simulink model "mrefrobotarm_modified_previous_y_previous_u_previous_ref_Thao"  (R2018b)
settings: Solver=FixedStepAuto  StartTime=0.0  StopTime=10  RelTol=1e-3  AbsTol=1e-6
undefined symbols (not defined in the file or in its folder): sfunxy2
libraries: neural x668, simulink x1
(part 17 of 21)

== system mrefrobotarm_modified_previous_y_previous_u_previous_ref_Thao/trimmed_cex/Layer 2/LW{2,1} ==
  "ad{2,1}" : Inport  PortDimensions=40
      mask Display: e = 0.06;c1 = [120 230 180]/255;c2 = ([120 230 180]+0)/(256+128);c3 = ([120 230 180]+128)/(256+128);patch([0 1 1 0],[0 0 1 1],c1);patch([0 1 1 1-e 1-e 0+e],[0 0 1 1-e 0+e 0+e],c2);patch([0 0 1 1-e 0+e 0+e],[0 1 1 1-e 1-e 0+e],c3);plot([0 1 1 0 0],[0 0 1 1 0]);
  "IW{2,1}(1,:)'" : Constant  Value=[-0.1197125311373569422901397274472401477396488189697265625;0.93141849603577753224925572794745676219463348388671875;0.004886359461366405858295802744351021829061210155487060546875;-0.1512746681304759643893476095399819314479827880859375;-0.167852357976244148662914312808425165712833404541015625;0.10006780281716527725155430061931838281452655792236328125;0.10181621299721650697467367763238144107162952423095703125;0.309725252258556238427189555295626632869243621826171875;-0.02933411195067354981791396539847482927143573760986328125;-0.0152198482308951478503278309517554589547216892242431640625;-0.330145430668005668284337161821895278990268707275390625;0.076789053257603046009904801394441165030002593994140625;-0.375398541974394428510919397012912668287754058837890625;0.382117841615298547974788334613549523055553436279296875;0.2201335081328267551104005406159558333456516265869140625;-0.13146013321116478689276618752046488225460052490234375;-0.0249539477614627684676218422055171686224639415740966796875;0.402936988611822866079847926812362857162952423095703125;-0.011171185980911817192673396448299172334372997283935546875;0.1036892109939195893986152441357262432575225830078125;-0.01468148224949680953621555801191789214499294757843017578125;-0.0351746242361976324541927851896616630256175994873046875;-0.45375320694342102800789007233106531202793121337890625;0.025604358260133124047808195200559566728770732879638671875;0.1991726441753766396747238331954577006399631500244140625;-0.19735600633120575775336646984214894473552703857421875;-0.0906818380815199720501595948007889091968536376953125;0.415050002351403268807672475304570980370044708251953125;0.2385038498913788773680977328695007599890232086181640625;0.053659262377953688416543087669197120703756809234619140625;-0.00831153444230189712704781612728766049258410930633544921875;-0.279703049728368624560204125373275019228458404541015625;-0.122675859787673591227985525620169937610626220703125;0.12231550321479693621551376736533711664378643035888671875;0.40279223208026382341273574638762511312961578369140625;0.398579712933626983950574640402919612824916839599609375;-0.0806627151487938343077388481106027029454708099365234375;0.262880682610419580402805195262772031128406524658203125;-0.73968018525003476071333352592773735523223876953125;-0.5854281940437520148634575889445841312408447265625]
      mask Display: e = 0.06;c1 = [120 150 230]/255;c2 = ([120 150 230]+0)/383;c3 = ([120 150 230]+128)/383;patch([0 1 1 0],[0 0 1 1],c1);patch([0 1 1 1-e 1-e 0+e],[0 0 1 1-e 0+e 0+e],c2);patch([0 0 1 1-e 0+e 0+e],[0 1 1 1-e 1-e 0+e],c3);plot([0 1 1 0 0],[0 0 1 1 0]);disp('weights');
  Mux : Mux  Inputs=1
      mask Display: e = 0.06;c1 = [120 150 230]/255;c2 = ([120 150 230]+0)/383;c3 = ([120 150 230]+128)/383;patch([0 1 1 0],[0 0 1 1],c1);patch([0 1 1 1-e 1-e 0+e],[0 0 1 1-e 0+e 0+e],c2);patch([0 0 1 1-e 0+e 0+e],[0 1 1 1-e 1-e 0+e],c3);plot([0 1 1 0 0],[0 0 1 1 0]);disp('Mux');
  dotprod1 : neural/Weight Functions/dotprod
  "lz{2,1}" : Outport
      mask Display: e = 0.06;c1 = [120 230 180]/255;c2 = ([120 230 180]+0)/(256+128);c3 = ([120 230 180]+128)/(256+128);patch([0 1 1 0],[0 0 1 1],c1);patch([0 1 1 1-e 1-e 0+e],[0 0 1 1-e 0+e 0+e],c2);patch([0 0 1 1-e 0+e 0+e],[0 1 1 1-e 1-e 0+e],c3);plot([0 1 1 0 0],[0 0 1 1 0]);
  wires:
  "IW{2,1}(1,:)'"/1 -> dotprod1/1
  "ad{2,1}"/1 -> dotprod1/2
  dotprod1/1 -> Mux/1
  Mux/1 -> "lz{2,1}"/1

== system mrefrobotarm_modified_previous_y_previous_u_previous_ref_Thao/trimmed_cex_2/Layer 1/Delays 1 ==
  "p{1}" : Inport  PortDimensions=10
      mask Display: e = 0.06;c1 = [120 230 180]/255;c2 = ([120 230 180]+0)/(256+128);c3 = ([120 230 180]+128)/(256+128);patch([0 1 1 0],[0 0 1 1],c1);patch([0 1 1 1-e 1-e 0+e],[0 0 1 1-e 0+e 0+e],c2);patch([0 0 1 1-e 0+e 0+e],[0 1 1 1-e 1-e 0+e],c3);plot([0 1 1 0 0],[0 0 1 1 0]);
  mux : Mux  Inputs=1
      mask Display: e = 0.06;c1 = [120 150 230]/255;c2 = ([120 150 230]+0)/383;c3 = ([120 150 230]+128)/383;patch([0 1 1 0],[0 0 1 1],c1);patch([0 1 1 1-e 1-e 0+e],[0 0 1 1-e 0+e 0+e],c2);patch([0 0 1 1-e 0+e 0+e],[0 1 1 1-e 1-e 0+e],c3);plot([0 1 1 0 0],[0 0 1 1 0]);disp('Mux')
  "pd{1,1}" : Outport
      mask Display: e = 0.06;c1 = [120 230 180]/255;c2 = ([120 230 180]+0)/(256+128);c3 = ([120 230 180]+128)/(256+128);patch([0 1 1 0],[0 0 1 1],c1);patch([0 1 1 1-e 1-e 0+e],[0 0 1 1-e 0+e 0+e],c2);patch([0 0 1 1-e 0+e 0+e],[0 1 1 1-e 1-e 0+e],c3);plot([0 1 1 0 0],[0 0 1 1 0]);
  wires:
  "p{1}"/1 -> mux/1
  mux/1 -> "pd{1,1}"/1

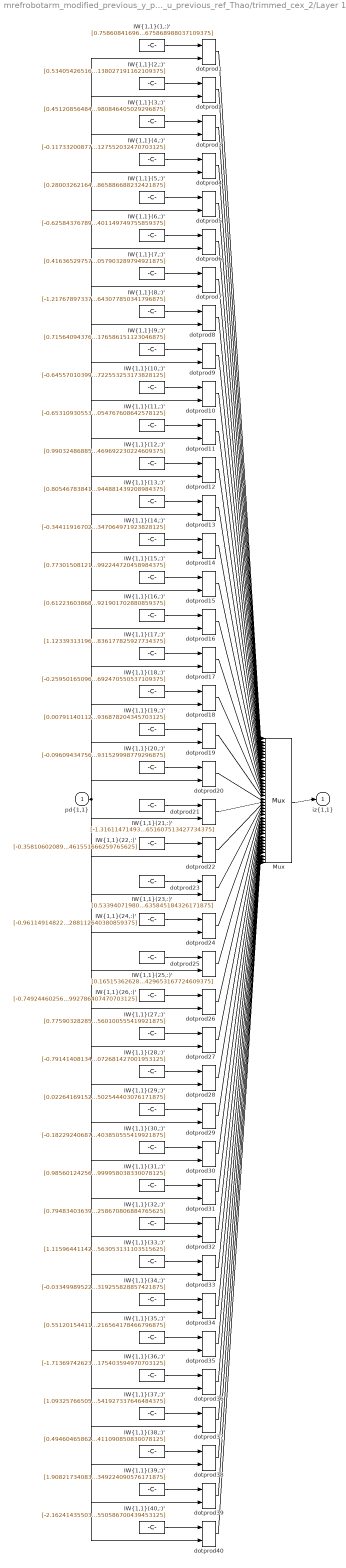
== system mrefrobotarm_modified_previous_y_previous_u_previous_ref_Thao/trimmed_cex_2/Layer 1/IW{1,1} ==
  "pd{1,1}" : Inport  PortDimensions=10
      mask Display: e = 0.06;c1 = [120 230 180]/255;c2 = ([120 230 180]+0)/(256+128);c3 = ([120 230 180]+128)/(256+128);patch([0 1 1 0],[0 0 1 1],c1);patch([0 1 1 1-e 1-e 0+e],[0 0 1 1-e 0+e 0+e],c2);patch([0 0 1 1-e 0+e 0+e],[0 1 1 1-e 1-e 0+e],c3);plot([0 1 1 0 0],[0 0 1 1 0]);
  "IW{1,1}(1,:)'" : Constant  Value=[0.7586084169638720453576752333901822566986083984375;0.64065528016229933427894138731062412261962890625;0.39576859169533984417199690142297185957431793212890625;0.67974231073814495029949966919957660138607025146484375;-0.8322839682529779015141002673772163689136505126953125;1.2325906050418289350290024231071583926677703857421875;-0.6476296846957207975492565310560166835784912109375;0.69513830019254607694989545052521862089633941650390625;0.362255404130632341352935554823488928377628326416015625;-0.83785018450818815605174449956393800675868988037109375]
      mask Display: e = 0.06;c1 = [120 150 230]/255;c2 = ([120 150 230]+0)/383;c3 = ([120 150 230]+128)/383;patch([0 1 1 0],[0 0 1 1],c1);patch([0 1 1 1-e 1-e 0+e],[0 0 1 1-e 0+e 0+e],c2);patch([0 0 1 1-e 0+e 0+e],[0 1 1 1-e 1-e 0+e],c3);plot([0 1 1 0 0],[0 0 1 1 0]);disp('Weights');
  "IW{1,1}(10,:)'" : Constant  Value=[-0.6455701039951160513652439476572908461093902587890625;0.6062395162995362074553895581630058586597442626953125;0.0841095892027095837217842699828906916081905364990234375;0.8395936116299094198467400929075665771961212158203125;-1.933433434291257579928924315026961266994476318359375;0.4699855661060308165133392321877181529998779296875;-1.3687077398461326982470609436859376728534698486328125;-0.1904722786551377999852974198802257888019084930419921875;0.326755886468258427424160572627442888915538787841796875;0.05237510702870014356324901427797158248722553253173828125]
      mask Display: e = 0.06;c1 = [120 150 230]/255;c2 = ([120 150 230]+0)/383;c3 = ([120 150 230]+128)/383;patch([0 1 1 0],[0 0 1 1],c1);patch([0 1 1 1-e 1-e 0+e],[0 0 1 1-e 0+e 0+e],c2);patch([0 0 1 1-e 0+e 0+e],[0 1 1 1-e 1-e 0+e],c3);plot([0 1 1 0 0],[0 0 1 1 0]);disp('Weights');
  "IW{1,1}(11,:)'" : Constant  Value=[-0.653109305534881112720313467434607446193695068359375;-0.63694471380195094578624548375955782830715179443359375;-0.66364616346480886921455066840280778706073760986328125;-1.5467933591431208828481658201781101524829864501953125;-0.953707704414698209660627981065772473812103271484375;0.016251165743796869289639062117203138768672943115234375;0.85764033268903105966529665238340385258197784423828125;-1.018200094286096923923423673841170966625213623046875;-1.006272936957347763353709524380974471569061279296875;-0.426306299052561066265099043448572047054767608642578125]
      mask Display: e = 0.06;c1 = [120 150 230]/255;c2 = ([120 150 230]+0)/383;c3 = ([120 150 230]+128)/383;patch([0 1 1 0],[0 0 1 1],c1);patch([0 1 1 1-e 1-e 0+e],[0 0 1 1-e 0+e 0+e],c2);patch([0 0 1 1-e 0+e 0+e],[0 1 1 1-e 1-e 0+e],c3);plot([0 1 1 0 0],[0 0 1 1 0]);disp('Weights');
  "IW{1,1}(12,:)'" : Constant  Value=[0.99032486885737236459448240566416643559932708740234375;-0.4064937633482277323793141476926393806934356689453125;-0.0653081845473883759733979559314320795238018035888671875;0.1267302228411903985971775910002179443836212158203125;-0.881843841858767074626257453928701579570770263671875;-0.062937554661245787013257313446956686675548553466796875;0.30167392474683563108328598900698125362396240234375;1.0408159785445139089432586843031458556652069091796875;-0.414501383489728036924049092704080976545810699462890625;-0.04337409273136037801688047466086572967469692230224609375]
      mask Display: e = 0.06;c1 = [120 150 230]/255;c2 = ([120 150 230]+0)/383;c3 = ([120 150 230]+128)/383;patch([0 1 1 0],[0 0 1 1],c1);patch([0 1 1 1-e 1-e 0+e],[0 0 1 1-e 0+e 0+e],c2);patch([0 0 1 1-e 0+e 0+e],[0 1 1 1-e 1-e 0+e],c3);plot([0 1 1 0 0],[0 0 1 1 0]);disp('Weights');
  "IW{1,1}(13,:)'" : Constant  Value=[0.80546783841772884304788249210105277597904205322265625;-0.0989022459644864071481862310974975116550922393798828125;-0.257406546599342422876333102976786904036998748779296875;-0.463638060984846667178516099738772027194499969482421875;0.118607183685509876003294493784778751432895660400390625;-1.064843433515526793797789650852791965007781982421875;-0.52909856619164463698012923487112857401371002197265625;-0.336660800704824236806445014735800214111804962158203125;-0.1735126677730877420291477619684883393347263336181640625;0.5562205162348961007268144385307095944881439208984375]
      mask Display: e = 0.06;c1 = [120 150 230]/255;c2 = ([120 150 230]+0)/383;c3 = ([120 150 230]+128)/383;patch([0 1 1 0],[0 0 1 1],c1);patch([0 1 1 1-e 1-e 0+e],[0 0 1 1-e 0+e 0+e],c2);patch([0 0 1 1-e 0+e 0+e],[0 1 1 1-e 1-e 0+e],c3);plot([0 1 1 0 0],[0 0 1 1 0]);disp('Weights');
  "IW{1,1}(14,:)'" : Constant  Value=[-0.344119167029077299702066738973371684551239013671875;-0.9444939814500035168975955457426607608795166015625;1.21324822037746482550346627249382436275482177734375;0.50228838522351237916296895491541363298892974853515625;0.3749062049519833461630469173542223870754241943359375;0.1968237635355130910053134130066609941422939300537109375;-0.33731776242260946840900714960298500955104827880859375;-0.1940053240678196733171034793485887348651885986328125;0.2162524161864634308916066629535635001957416534423828125;-0.58841906490396056472746977306087501347064971923828125]
      mask Display: e = 0.06;c1 = [120 150 230]/255;c2 = ([120 150 230]+0)/383;c3 = ([120 150 230]+128)/383;patch([0 1 1 0],[0 0 1 1],c1);patch([0 1 1 1-e 1-e 0+e],[0 0 1 1-e 0+e 0+e],c2);patch([0 0 1 1-e 0+e 0+e],[0 1 1 1-e 1-e 0+e],c3);plot([0 1 1 0 0],[0 0 1 1 0]);disp('Weights');
  "IW{1,1}(15,:)'" : Constant  Value=[0.773015081210556065371974909794516861438751220703125;-0.214501050742608112553710952852270565927028656005859375;0.058329420791091650400073120863453368656337261199951171875;-1.0031154839416005497554351677536033093929290771484375;-0.4021214748246746406579177346429787576198577880859375;1.0874132509379077493605336712789721786975860595703125;0.47867402206187625868238910697982646524906158447265625;0.279250200051134100931449211202561855316162109375;-0.65106152721032650720900392116163857281208038330078125;0.53527506313622497113868803353398106992244720458984375]
      mask Display: e = 0.06;c1 = [120 150 230]/255;c2 = ([120 150 230]+0)/383;c3 = ([120 150 230]+128)/383;patch([0 1 1 0],[0 0 1 1],c1);patch([0 1 1 1-e 1-e 0+e],[0 0 1 1-e 0+e 0+e],c2);patch([0 0 1 1-e 0+e 0+e],[0 1 1 1-e 1-e 0+e],c3);plot([0 1 1 0 0],[0 0 1 1 0]);disp('Weights');
  "IW{1,1}(16,:)'" : Constant  Value=[0.61223603868116993620418497812352143228054046630859375;-0.438972085640134179751470355768105946481227874755859375;-0.3260916742501061005299334283336065709590911865234375;0.314454773325576864007047106497338972985744476318359375;-0.7703308680068090552595094777643680572509765625;-0.07077459320376415508047074354180949740111827850341796875;1.24224649787842356118972020340152084827423095703125;-0.70133690239806545374534607617533765733242034912109375;-0.6441671392670060836138645754544995725154876708984375;-1.4524212049430287319040644433698616921901702880859375]
      mask Display: e = 0.06;c1 = [120 150 230]/255;c2 = ([120 150 230]+0)/383;c3 = ([120 150 230]+128)/383;patch([0 1 1 0],[0 0 1 1],c1);patch([0 1 1 1-e 1-e 0+e],[0 0 1 1-e 0+e 0+e],c2);patch([0 0 1 1-e 0+e 0+e],[0 1 1 1-e 1-e 0+e],c3);plot([0 1 1 0 0],[0 0 1 1 0]);disp('Weights');
  "IW{1,1}(17,:)'" : Constant  Value=[1.1233931319610797050501105331932194530963897705078125;-0.78936101311700446192531899214372970163822174072265625;0.49335086052196885919585156443645246326923370361328125;-0.94507727258668883241199409894761629402637481689453125;-0.91975779633484833208711961560766212642192840576171875;-0.02441081487389241966301511865822249092161655426025390625;-0.433851875953729149149040722477366216480731964111328125;-0.592411984412089420715119558735750615596771240234375;0.3930137097113084454491627184324897825717926025390625;0.63257120943745570595950766801252029836177825927734375]
      mask Display: e = 0.06;c1 = [120 150 230]/255;c2 = ([120 150 230]+0)/383;c3 = ([120 150 230]+128)/383;patch([0 1 1 0],[0 0 1 1],c1);patch([0 1 1 1-e 1-e 0+e],[0 0 1 1-e 0+e 0+e],c2);patch([0 0 1 1-e 0+e 0+e],[0 1 1 1-e 1-e 0+e],c3);plot([0 1 1 0 0],[0 0 1 1 0]);disp('Weights');
  "IW{1,1}(18,:)'" : Constant  Value=[-0.259501650964344243721626526166801340878009796142578125;-0.8925682730605697390302566418540664017200469970703125;0.21119409423119150925884923708508722484111785888671875;-0.020242270458488594020440842768948641605675220489501953125;0.221870071791709033703909881296567618846893310546875;1.005093632581294027517060385434888303279876708984375;-0.1912291311650022862522746436297893524169921875;0.74135343706830825194487033513723872601985931396484375;1.190527999679797943599623977206647396087646484375;-0.395164188059986931644829155629849992692470550537109375]
      mask Display: e = 0.06;c1 = [120 150 230]/255;c2 = ([120 150 230]+0)/383;c3 = ([120 150 230]+128)/383;patch([0 1 1 0],[0 0 1 1],c1);patch([0 1 1 1-e 1-e 0+e],[0 0 1 1-e 0+e 0+e],c2);patch([0 0 1 1-e 0+e 0+e],[0 1 1 1-e 1-e 0+e],c3);plot([0 1 1 0 0],[0 0 1 1 0]);disp('Weights');
  "IW{1,1}(19,:)'" : Constant  Value=[0.00791140112843116173613200459158179000951349735260009765625;-0.346856168232712980259435653351829387247562408447265625;-0.90950554322576537824573961188434623181819915771484375;0.5507910617541040831923737641773186624050140380859375;0.2808732150432777796567052064347080886363983154296875;0.7225570652344941446898474168847315013408660888671875;0.207719295598636055633079422477749176323413848876953125;0.8557900847635668828417010445264168083667755126953125;0.1488913455577660638340375953703187406063079833984375;0.93406442221251151369898479970288462936878204345703125]
      mask Display: e = 0.06;c1 = [120 150 230]/255;c2 = ([120 150 230]+0)/383;c3 = ([120 150 230]+128)/383;patch([0 1 1 0],[0 0 1 1],c1);patch([0 1 1 1-e 1-e 0+e],[0 0 1 1-e 0+e 0+e],c2);patch([0 0 1 1-e 0+e 0+e],[0 1 1 1-e 1-e 0+e],c3);plot([0 1 1 0 0],[0 0 1 1 0]);disp('Weights');
  "IW{1,1}(2,:)'" : Constant  Value=[0.5340542651614705871310206930502317845821380615234375;-0.50044840681500313284146841397159732878208160400390625;0.74098040354179806055157087030238471925258636474609375;0.69217188016377739767648336055572144687175750732421875;1.05191904124650914553740221890620887279510498046875;0.8046954420890168879765269593917764723300933837890625;-0.07378431287153304485304516902033356018364429473876953125;1.164405197692230498063281629583798348903656005859375;0.337370058157611063531788886393769644200801849365234375;0.499213183565015261589081774218357168138027191162109375]
      mask Display: e = 0.06;c1 = [120 150 230]/255;c2 = ([120 150 230]+0)/383;c3 = ([120 150 230]+128)/383;patch([0 1 1 0],[0 0 1 1],c1);patch([0 1 1 1-e 1-e 0+e],[0 0 1 1-e 0+e 0+e],c2);patch([0 0 1 1-e 0+e 0+e],[0 1 1 1-e 1-e 0+e],c3);plot([0 1 1 0 0],[0 0 1 1 0]);disp('Weights');
  "IW{1,1}(20,:)'" : Constant  Value=[-0.09609434756546129940968370419795974157750606536865234375;0.19673535843828826585877322941087186336517333984375;0.485082405139408201488748773044790141284465789794921875;0.3015027352977599495176264099427498877048492431640625;-0.80194218391999694262040065950714051723480224609375;0.5184479332624924996508752883528359234333038330078125;-0.63167627182296814947193297484773211181163787841796875;-0.717734118866697912153540528379380702972412109375;-0.1995948861736938917399442061650916002690792083740234375;-0.288686266459039220233506739532458595931529998779296875]
      mask Display: e = 0.06;c1 = [120 150 230]/255;c2 = ([120 150 230]+0)/383;c3 = ([120 150 230]+128)/383;patch([0 1 1 0],[0 0 1 1],c1);patch([0 1 1 1-e 1-e 0+e],[0 0 1 1-e 0+e 0+e],c2);patch([0 0 1 1-e 0+e 0+e],[0 1 1 1-e 1-e 0+e],c3);plot([0 1 1 0 0],[0 0 1 1 0]);disp('Weights');
  "IW{1,1}(21,:)'" : Constant  Value=[-1.316114714930880946752722593373619019985198974609375;-0.391331914698053784373854568912065587937831878662109375;1.255126089641885211989347226335667073726654052734375;0.053082231395421751452001757343168719671666622161865234375;-0.370186780392510572657016609809943474829196929931640625;0.42184518923261926648393682626192457973957061767578125;0.313647539459381896609357909255777485668659210205078125;0.64087383210082704554366728189052082598209381103515625;0.28799774286481161222894797901972196996212005615234375;1.578823148278269083988334386958740651607513427734375]
      mask Display: e = 0.06;c1 = [120 150 230]/255;c2 = ([120 150 230]+0)/383;c3 = ([120 150 230]+128)/383;patch([0 1 1 0],[0 0 1 1],c1);patch([0 1 1 1-e 1-e 0+e],[0 0 1 1-e 0+e 0+e],c2);patch([0 0 1 1-e 0+e 0+e],[0 1 1 1-e 1-e 0+e],c3);plot([0 1 1 0 0],[0 0 1 1 0]);disp('Weights');
  "IW{1,1}(22,:)'" : Constant  Value=[-0.358106020899803978441156004919321276247501373291015625;-1.2655593113213015055151799970190040767192840576171875;-0.558671247763788070272994445986114442348480224609375;-0.66943569832340477088195029864436946809291839599609375;-1.7087344935301966852847499467316083610057830810546875;0.8904147532676358611780642604571767151355743408203125;0.10252753796185477830338328431025729514658451080322265625;-1.4094656324850813877702648824197240173816680908203125;-0.387970281202749844862154304792056791484355926513671875;0.254687717231173726961657166611985303461551666259765625]
      mask Display: e = 0.06;c1 = [120 150 230]/255;c2 = ([120 150 230]+0)/383;c3 = ([120 150 230]+128)/383;patch([0 1 1 0],[0 0 1 1],c1);patch([0 1 1 1-e 1-e 0+e],[0 0 1 1-e 0+e 0+e],c2);patch([0 0 1 1-e 0+e 0+e],[0 1 1 1-e 1-e 0+e],c3);plot([0 1 1 0 0],[0 0 1 1 0]);disp('Weights');
  "IW{1,1}(23,:)'" : Constant  Value=[0.53394071980779056474375465768389403820037841796875;-0.097326372325129140161692475885502062737941741943359375;0.394713326811878262301291897529154084622859954833984375;-0.77411496543627145161536873274599201977252960205078125;-0.75735432012757553099646656846744008362293243408203125;0.50212897318520022249543899306445382535457611083984375;0.53375092830104831076454274807474575936794281005859375;-0.81041995022959412153795710764825344085693359375;-0.9361788723115889165882208544644527137279510498046875;0.397958513870448893356979169766418635845184326171875]
      mask Display: e = 0.06;c1 = [120 150 230]/255;c2 = ([120 150 230]+0)/383;c3 = ([120 150 230]+128)/383;patch([0 1 1 0],[0 0 1 1],c1);patch([0 1 1 1-e 1-e 0+e],[0 0 1 1-e 0+e 0+e],c2);patch([0 0 1 1-e 0+e 0+e],[0 1 1 1-e 1-e 0+e],c3);plot([0 1 1 0 0],[0 0 1 1 0]);disp('Weights');
  "IW{1,1}(24,:)'" : Constant  Value=[-0.96114914822197761168354190886020660400390625;0.310068469178645778061564897143398411571979522705078125;-0.52287237915203832461230604167212732136249542236328125;-0.46518339424300803042200413983664475381374359130859375;-0.65401684243875701785242426922195591032505035400390625;0.7290250379247746881361535997712053358554840087890625;1.1985462246318212553575222045765258371829986572265625;-0.89713817604706524999613748150295577943325042724609375;0.23287611745276881602961793760186992585659027099609375;0.1302666056399977845270399257060489617288112640380859375]
      mask Display: e = 0.06;c1 = [120 150 230]/255;c2 = ([120 150 230]+0)/383;c3 = ([120 150 230]+128)/383;patch([0 1 1 0],[0 0 1 1],c1);patch([0 1 1 1-e 1-e 0+e],[0 0 1 1-e 0+e 0+e],c2);patch([0 0 1 1-e 0+e 0+e],[0 1 1 1-e 1-e 0+e],c3);plot([0 1 1 0 0],[0 0 1 1 0]);disp('Weights');
  "IW{1,1}(25,:)'" : Constant  Value=[0.165153626284937071755365423086914233863353729248046875;-0.052135775738207316976069449765418539755046367645263671875;0.77373592515846090211795171853736974298954010009765625;0.98452216342932530324105755425989627838134765625;-2.551215629798953887785728511516936123371124267578125;-0.11003524514953545720974403820946463383734226226806640625;-0.10410308600901836684204937455433537252247333526611328125;-0.6754741305758014124904775599134154617786407470703125;-0.08721343582435410468622905000302125699818134307861328125;0.601485088117703181609385865158401429653167724609375]
      mask Display: e = 0.06;c1 = [120 150 230]/255;c2 = ([120 150 230]+0)/383;c3 = ([120 150 230]+128)/383;patch([0 1 1 0],[0 0 1 1],c1);patch([0 1 1 1-e 1-e 0+e],[0 0 1 1-e 0+e 0+e],c2);patch([0 0 1 1-e 0+e 0+e],[0 1 1 1-e 1-e 0+e],c3);plot([0 1 1 0 0],[0 0 1 1 0]);disp('Weights');
  "IW{1,1}(26,:)'" : Constant  Value=[-0.74924460256466918206541549807297997176647186279296875;-0.36294009921175440780416465713642537593841552734375;-0.76862280998369281181936685243272222578525543212890625;-1.237638376690007202540755315567366778850555419921875;0.07000727279722600282507727342817815952003002166748046875;0.613374495092073868107718226383440196514129638671875;-0.439395209787314333649277386939502321183681488037109375;-0.456194981024637957744971572537906467914581298828125;-0.6359836310345177157188345518079586327075958251953125;-0.65551421356994776790116929987561888992786407470703125]
      mask Display: e = 0.06;c1 = [120 150 230]/255;c2 = ([120 150 230]+0)/383;c3 = ([120 150 230]+128)/383;patch([0 1 1 0],[0 0 1 1],c1);patch([0 1 1 1-e 1-e 0+e],[0 0 1 1-e 0+e 0+e],c2);patch([0 0 1 1-e 0+e 0+e],[0 1 1 1-e 1-e 0+e],c3);plot([0 1 1 0 0],[0 0 1 1 0]);disp('Weights');
  "IW{1,1}(27,:)'" : Constant  Value=[0.77590328285638410221736194216646254062652587890625;0.08179991836539689253893214981872006319463253021240234375;0.6728716128491820658297228874289430677890777587890625;-0.420053163988742206402804413301055319607257843017578125;1.1608908802335788923443260500789619982242584228515625;-0.42788666442380296484060409056837670505046844482421875;0.359136746250959426607352042992715723812580108642578125;0.85427140533849066361682389469933696091175079345703125;-0.4412316264510287577849112494732253253459930419921875;-0.78149847422082963088740825696731917560100555419921875]
      mask Display: e = 0.06;c1 = [120 150 230]/255;c2 = ([120 150 230]+0)/383;c3 = ([120 150 230]+128)/383;patch([0 1 1 0],[0 0 1 1],c1);patch([0 1 1 1-e 1-e 0+e],[0 0 1 1-e 0+e 0+e],c2);patch([0 0 1 1-e 0+e 0+e],[0 1 1 1-e 1-e 0+e],c3);plot([0 1 1 0 0],[0 0 1 1 0]);disp('Weights');
  "IW{1,1}(28,:)'" : Constant  Value=[-0.7914140813487595682573783051338978111743927001953125;0.222136642111575743907536661936319433152675628662109375;-1.0729904368246945267628689180128276348114013671875;-0.2498907225014191657574968985500163398683071136474609375;0.62388770080220290470407462635193951427936553955078125;0.242381202805197870642217594649991951882839202880859375;-0.03781574301987257469281900057467282749712467193603515625;-1.09711242046527868154726093052886426448822021484375;0.645894038787806490375942303217016160488128662109375;1.2553168854993803638109284293022938072681427001953125]
      mask Display: e = 0.06;c1 = [120 150 230]/255;c2 = ([120 150 230]+0)/383;c3 = ([120 150 230]+128)/383;patch([0 1 1 0],[0 0 1 1],c1);patch([0 1 1 1-e 1-e 0+e],[0 0 1 1-e 0+e 0+e],c2);patch([0 0 1 1-e 0+e 0+e],[0 1 1 1-e 1-e 0+e],c3);plot([0 1 1 0 0],[0 0 1 1 0]);disp('Weights');
  "IW{1,1}(29,:)'" : Constant  Value=[0.022641691527972740427543385521857999265193939208984375;-0.406312170753067636308486498819547705352306365966796875;0.24032865868175823376162725253379903733730316162109375;-0.1444131097323844981072937798671773634850978851318359375;-0.84026770861194466366583810668089427053928375244140625;-0.82185563415251416952145291361375711858272552490234375;-0.476662772527611522388468756616930477321147918701171875;0.6146644261520222141115254999021999537944793701171875;-1.3988170673402020582898330758325755596160888671875;0.06328824692809935370529927922689239494502544403076171875]
      mask Display: e = 0.06;c1 = [120 150 230]/255;c2 = ([120 150 230]+0)/383;c3 = ([120 150 230]+128)/383;patch([0 1 1 0],[0 0 1 1],c1);patch([0 1 1 1-e 1-e 0+e],[0 0 1 1-e 0+e 0+e],c2);patch([0 0 1 1-e 0+e 0+e],[0 1 1 1-e 1-e 0+e],c3);plot([0 1 1 0 0],[0 0 1 1 0]);disp('Weights');
  "IW{1,1}(3,:)'" : Constant  Value=[0.451208564841975301451526547680259682238101959228515625;0.814033236546007454847995177260600030422210693359375;1.262153046410520840225899519282393157482147216796875;0.78879689292423871282977643204503692686557769775390625;0.92884958479045176549249163144850172102451324462890625;-0.27833656486401003871122838972951285541057586669921875;1.1598080641425172476743910010554827749729156494140625;-0.1849418287742990163469158915177104063332080841064453125;-0.88037331169577814904414481134153902530670166015625;0.26887773273454829148221278956043533980846405029296875]
      mask Display: e = 0.06;c1 = [120 150 230]/255;c2 = ([120 150 230]+0)/383;c3 = ([120 150 230]+128)/383;patch([0 1 1 0],[0 0 1 1],c1);patch([0 1 1 1-e 1-e 0+e],[0 0 1 1-e 0+e 0+e],c2);patch([0 0 1 1-e 0+e 0+e],[0 1 1 1-e 1-e 0+e],c3);plot([0 1 1 0 0],[0 0 1 1 0]);disp('Weights');
  "IW{1,1}(30,:)'" : Constant  Value=[-0.18229240687955450272994539773208089172840118408203125;0.85925362669036975393765942499157972633838653564453125;0.72086939041646524994888522996916435658931732177734375;0.1540456983739212082351599519824958406388759613037109375;-0.87905145148783170316875157368485815823078155517578125;0.64648266484036087664577507894136942923069000244140625;0.31664040001570736837521735651534982025623321533203125;0.2472269665495660795340171489442582242190837860107421875;0.5162714411272750769654749092296697199344635009765625;-0.4047857135702066511129260106827132403850555419921875]
      mask Display: e = 0.06;c1 = [120 150 230]/255;c2 = ([120 150 230]+0)/383;c3 = ([120 150 230]+128)/383;patch([0 1 1 0],[0 0 1 1],c1);patch([0 1 1 1-e 1-e 0+e],[0 0 1 1-e 0+e 0+e],c2);patch([0 0 1 1-e 0+e 0+e],[0 1 1 1-e 1-e 0+e],c3);plot([0 1 1 0 0],[0 0 1 1 0]);disp('Weights');
  "IW{1,1}(31,:)'" : Constant  Value=[0.98560124256052883406908904362353496253490447998046875;-0.2284442932273070547832816146183176897466182708740234375;0.61461825619302157264201014186255633831024169921875;-0.54626893543429655419885193623485974967479705810546875;-1.1005059758909154776773675621370784938335418701171875;-1.15525185722439882596290772198699414730072021484375;-0.1398693596401139604967767127163824625313282012939453125;-0.74888072834453944803811964447959326207637786865234375;-0.53986343200050324053762551557156257331371307373046875;0.95215527816649647707691883624647743999958038330078125]
      mask Display: e = 0.06;c1 = [120 150 230]/255;c2 = ([120 150 230]+0)/383;c3 = ([120 150 230]+128)/383;patch([0 1 1 0],[0 0 1 1],c1);patch([0 1 1 1-e 1-e 0+e],[0 0 1 1-e 0+e 0+e],c2);patch([0 0 1 1-e 0+e 0+e],[0 1 1 1-e 1-e 0+e],c3);plot([0 1 1 0 0],[0 0 1 1 0]);disp('Weights');
  "IW{1,1}(32,:)'" : Constant  Value=[0.79483403639315619582106364759965799748897552490234375;-0.266092993127061472335981306969188153743743896484375;1.2827148241728905109226843705982901155948638916015625;0.1202392401203307426005295610593748278915882110595703125;0.378744828732331340059857893720618449151515960693359375;1.1608692265820568234602205848204903304576873779296875;0.596714276467414261873045688844285905361175537109375;0.70573427243436570588386302915751002728939056396484375;-0.24178744837182886140425353005412034690380096435546875;0.93079293772478044477480807472602464258670806884765625]
      mask Display: e = 0.06;c1 = [120 150 230]/255;c2 = ([120 150 230]+0)/383;c3 = ([120 150 230]+128)/383;patch([0 1 1 0],[0 0 1 1],c1);patch([0 1 1 1-e 1-e 0+e],[0 0 1 1-e 0+e 0+e],c2);patch([0 0 1 1-e 0+e 0+e],[0 1 1 1-e 1-e 0+e],c3);plot([0 1 1 0 0],[0 0 1 1 0]);disp('Weights');
  "IW{1,1}(33,:)'" : Constant  Value=[1.1159644114215196974981836319784633815288543701171875;-1.4094635911002715289441766799427568912506103515625;-0.63434533907462997692761064172373153269290924072265625;-0.20731565618138458884089914135984145104885101318359375;1.6711002605418967537076468943268992006778717041015625;-0.30502988545126130670581687809317372739315032958984375;-0.353718916889357526400772258057259023189544677734375;0.43956458172074575063703605337650515139102935791015625;0.024052669154595855693923311946491594426333904266357421875;0.67409393540274165079750900986255146563053131103515625]
      mask Display: e = 0.06;c1 = [120 150 230]/255;c2 = ([120 150 230]+0)/383;c3 = ([120 150 230]+128)/383;patch([0 1 1 0],[0 0 1 1],c1);patch([0 1 1 1-e 1-e 0+e],[0 0 1 1-e 0+e 0+e],c2);patch([0 0 1 1-e 0+e 0+e],[0 1 1 1-e 1-e 0+e],c3);plot([0 1 1 0 0],[0 0 1 1 0]);disp('Weights');
  "IW{1,1}(34,:)'" : Constant  Value=[-0.033499895221541294010325628960345056839287281036376953125;1.8336900610781279308270086403354071080684661865234375;0.99092194457313331756864727140055038034915924072265625;1.2945525785874867352731598657555878162384033203125;0.139409344368469245711850135194254107773303985595703125;0.393311905574143694241939783751149661839008331298828125;0.270480232146603161158537886876729317009449005126953125;-0.0967684878388183900010943716551992110908031463623046875;-0.50659479936684326251139509622589685022830963134765625;-0.35639814861579643956446261654491536319255828857421875]
      mask Display: e = 0.06;c1 = [120 150 230]/255;c2 = ([120 150 230]+0)/383;c3 = ([120 150 230]+128)/383;patch([0 1 1 0],[0 0 1 1],c1);patch([0 1 1 1-e 1-e 0+e],[0 0 1 1-e 0+e 0+e],c2);patch([0 0 1 1-e 0+e 0+e],[0 1 1 1-e 1-e 0+e],c3);plot([0 1 1 0 0],[0 0 1 1 0]);disp('Weights');
  "IW{1,1}(35,:)'" : Constant  Value=[0.551201544111604935238801772356964647769927978515625;-0.450089054283685452428898088328423909842967987060546875;-0.251368395564277091747129588839015923440456390380859375;-0.2772400638463474731310043353005312383174896240234375;1.4398978848694667931340518407523632049560546875;0.9574023193422409594433020174619741737842559814453125;0.96095613233503396344303837395273149013519287109375;-0.467717984755913251948555853232392109930515289306640625;0.90978462471178123127657499935594387352466583251953125;0.8450144208930925326939131991821341216564178466796875]
      mask Display: e = 0.06;c1 = [120 150 230]/255;c2 = ([120 150 230]+0)/383;c3 = ([120 150 230]+128)/383;patch([0 1 1 0],[0 0 1 1],c1);patch([0 1 1 1-e 1-e 0+e],[0 0 1 1-e 0+e 0+e],c2);patch([0 0 1 1-e 0+e 0+e],[0 1 1 1-e 1-e 0+e],c3);plot([0 1 1 0 0],[0 0 1 1 0]);disp('Weights');
  "IW{1,1}(36,:)'" : Constant  Value=[-1.7136974262307427263607451095595024526119232177734375;0.78994076973646409900453591035329736769199371337890625;0.52361808850390101355287697515450417995452880859375;-0.293086328535619167201531354294274933636188507080078125;0.1818749290196476631198407858391874469816684722900390625;-0.1732686383786937456275012436890392564237117767333984375;-0.498256048276367435878597689224989153444766998291015625;0.96794984944336814880472275035572238266468048095703125;-0.3339666743480240729269326038775034248828887939453125;-0.7002849026877495663967465588939376175403594970703125]
      mask Display: e = 0.06;c1 = [120 150 230]/255;c2 = ([120 150 230]+0)/383;c3 = ([120 150 230]+128)/383;patch([0 1 1 0],[0 0 1 1],c1);patch([0 1 1 1-e 1-e 0+e],[0 0 1 1-e 0+e 0+e],c2);patch([0 0 1 1-e 0+e 0+e],[0 1 1 1-e 1-e 0+e],c3);plot([0 1 1 0 0],[0 0 1 1 0]);disp('Weights');
  "IW{1,1}(37,:)'" : Constant  Value=[1.09325766505933952288387445150874555110931396484375;0.5842526023513838762113437041989527642726898193359375;-0.251848528617412414920551100294687785208225250244140625;1.213611038066297442838958886568434536457061767578125;0.251448565862028183826026861424907110631465911865234375;0.56850361478417033023191606844193302094936370849609375;0.794047191398292273589731848915107548236846923828125;0.89893395461028957615923218327225185930728912353515625;0.63277524871377910375969122469541616737842559814453125;-0.88669898822682480243884128867648541927337646484375]
      mask Display: e = 0.06;c1 = [120 150 230]/255;c2 = ([120 150 230]+0)/383;c3 = ([120 150 230]+128)/383;patch([0 1 1 0],[0 0 1 1],c1);patch([0 1 1 1-e 1-e 0+e],[0 0 1 1-e 0+e 0+e],c2);patch([0 0 1 1-e 0+e 0+e],[0 1 1 1-e 1-e 0+e],c3);plot([0 1 1 0 0],[0 0 1 1 0]);disp('Weights');
  "IW{1,1}(38,:)'" : Constant  Value=[0.4946046586293018076929683957132510840892791748046875;-1.1599243422025347083348378873779438436031341552734375;0.12457441384673202666721891773704555816948413848876953125;-0.6213377944132558727829973577172495424747467041015625;-0.3298729627729024560522930187289603054523468017578125;0.64504375115380663263664473561220802366733551025390625;-1.3394013608609960375162017953698523342609405517578125;-0.59228693578657687357491568036493845283985137939453125;0.478517131561791597693655830880743451416492462158203125;-1.1671517341768400388701820702408440411090850830078125]
      mask Display: e = 0.06;c1 = [120 150 230]/255;c2 = ([120 150 230]+0)/383;c3 = ([120 150 230]+128)/383;patch([0 1 1 0],[0 0 1 1],c1);patch([0 1 1 1-e 1-e 0+e],[0 0 1 1-e 0+e 0+e],c2);patch([0 0 1 1-e 0+e 0+e],[0 1 1 1-e 1-e 0+e],c3);plot([0 1 1 0 0],[0 0 1 1 0]);disp('Weights');
  "IW{1,1}(39,:)'" : Constant  Value=[1.9082173408328884089968369153211824595928192138671875;0.05572851562233428757142661424950347281992435455322265625;0.39614735715188353903926099519594572484493255615234375;0.9543446984192487381193359397002495825290679931640625;0.7743781805223501901735971841844730079174041748046875;0.22253234642159147593787338337278924882411956787109375;0.74003249681866434261934273308725096285343170166015625;0.312908128488276926493227847458911128342151641845703125;0.184697618337192281945391414410551078617572784423828125;0.055787807238861834846499476725512067787349224090576171875]
      mask Display: e = 0.06;c1 = [120 150 230]/255;c2 = ([120 150 230]+0)/383;c3 = ([120 150 230]+128)/383;patch([0 1 1 0],[0 0 1 1],c1);patch([0 1 1 1-e 1-e 0+e],[0 0 1 1-e 0+e 0+e],c2);patch([0 0 1 1-e 0+e 0+e],[0 1 1 1-e 1-e 0+e],c3);plot([0 1 1 0 0],[0 0 1 1 0]);disp('Weights');
  "IW{1,1}(4,:)'" : Constant  Value=[-0.1173320087750106266444305447294027544558048248291015625;1.3480670350617087738243071726174093782901763916015625;-0.354705902679712192782091051412862725555896759033203125;0.77333861363924294440863604904734529554843902587890625;1.63579225791282656388148097903467714786529541015625;-0.11123350434094932126516397374871303327381610870361328125;0.5482823462094066346850240734056569635868072509765625;0.1402281943298513688933581988749210722744464874267578125;0.0867282551135314661028274940690607763826847076416015625;0.5414561817666279086580516377580352127552032470703125]
      mask Display: e = 0.06;c1 = [120 150 230]/255;c2 = ([120 150 230]+0)/383;c3 = ([120 150 230]+128)/383;patch([0 1 1 0],[0 0 1 1],c1);patch([0 1 1 1-e 1-e 0+e],[0 0 1 1-e 0+e 0+e],c2);patch([0 0 1 1-e 0+e 0+e],[0 1 1 1-e 1-e 0+e],c3);plot([0 1 1 0 0],[0 0 1 1 0]);disp('Weights');
  "IW{1,1}(40,:)'" : Constant  Value=[-2.162414355031302193310693837702274322509765625;-1.2173220305798848617229168667108751833438873291015625;-1.069471709653666113837289231014437973499298095703125;-0.72243897356051489655470732031972147524356842041015625;-0.2327708426346479786417376089957542717456817626953125;-1.0722705845581808059563400092883966863155364990234375;-0.8674279942641993645935372114763595163822174072265625;-2.233540487559733112021831402671523392200469970703125;-0.367618008133395957059974534786306321620941162109375;-0.6475618079486100686636973478016443550586700439453125]
      mask Display: e = 0.06;c1 = [120 150 230]/255;c2 = ([120 150 230]+0)/383;c3 = ([120 150 230]+128)/383;patch([0 1 1 0],[0 0 1 1],c1);patch([0 1 1 1-e 1-e 0+e],[0 0 1 1-e 0+e 0+e],c2);patch([0 0 1 1-e 0+e 0+e],[0 1 1 1-e 1-e 0+e],c3);plot([0 1 1 0 0],[0 0 1 1 0]);disp('Weights');
  "IW{1,1}(5,:)'" : Constant  Value=[0.280032621644622725654016903718002140522003173828125;0.31162674470934048631676205332041718065738677978515625;0.73329444838142432416816518525592982769012451171875;-0.74381831507047435625423759120167233049869537353515625;-0.2037431421778120033128089971796725876629352569580078125;-0.216666483780353524846162827088846825063228607177734375;0.83956626956612512291400207686820067465305328369140625;0.10346669895444744746715315386609290726482868194580078125;-0.48817944431931448168171527868253178894519805908203125;-1.314565311635582656180076810414902865886688232421875]
      mask Display: e = 0.06;c1 = [120 150 230]/255;c2 = ([120 150 230]+0)/383;c3 = ([120 150 230]+128)/383;patch([0 1 1 0],[0 0 1 1],c1);patch([0 1 1 1-e 1-e 0+e],[0 0 1 1-e 0+e 0+e],c2);patch([0 0 1 1-e 0+e 0+e],[0 1 1 1-e 1-e 0+e],c3);plot([0 1 1 0 0],[0 0 1 1 0]);disp('Weights');
  "IW{1,1}(6,:)'" : Constant  Value=[-0.62584376789803985996485380383091978728771209716796875;-0.540032257019178896229050224064849317073822021484375;-0.81057890967026946515971985718351788818836212158203125;-0.71273580315754514469261948761413805186748504638671875;0.28461546439817320131027145180269144475460052490234375;-0.6550068298352347273549867168185301125049591064453125;-0.5546141171316401052848732433631084859371185302734375;-1.1037070954587704374461054612766019999980926513671875;0.07804229967168128945242955296635045669972896575927734375;0.363107460042218332940677782971761189401149749755859375]
      mask Display: e = 0.06;c1 = [120 150 230]/255;c2 = ([120 150 230]+0)/383;c3 = ([120 150 230]+128)/383;patch([0 1 1 0],[0 0 1 1],c1);patch([0 1 1 1-e 1-e 0+e],[0 0 1 1-e 0+e 0+e],c2);patch([0 0 1 1-e 0+e 0+e],[0 1 1 1-e 1-e 0+e],c3);plot([0 1 1 0 0],[0 0 1 1 0]);disp('Weights');
  "IW{1,1}(7,:)'" : Constant  Value=[0.416365297579853577136788089774199761450290679931640625;-0.56943299777566080965840455974102951586246490478515625;0.57493518434140533646115045485203154385089874267578125;0.64415606893323740234080787558923475444316864013671875;-0.2153918058795817602746325292173423804342746734619140625;0.347216008767543049540194033397710882127285003662109375;-0.1431779117060572037445353998919017612934112548828125;0.8481090788288891957336090854369103908538818359375;-0.830628524455353289823733575758524239063262939453125;1.007356102126159225207402414525859057903289794921875]
      mask Display: e = 0.06;c1 = [120 150 230]/255;c2 = ([120 150 230]+0)/383;c3 = ([120 150 230]+128)/383;patch([0 1 1 0],[0 0 1 1],c1);patch([0 1 1 1-e 1-e 0+e],[0 0 1 1-e 0+e 0+e],c2);patch([0 0 1 1-e 0+e 0+e],[0 1 1 1-e 1-e 0+e],c3);plot([0 1 1 0 0],[0 0 1 1 0]);disp('Weights');
  "IW{1,1}(8,:)'" : Constant  Value=[-1.217678973372162243293814753997139632701873779296875;-0.049744915705065791133865360507115838117897510528564453125;0.99468321524782654652341307155438698828220367431640625;1.3871077805052800524521217084839008748531341552734375;-0.1080317006413676061971074204848264344036579132080078125;0.309627070800922610249727995324064977467060089111328125;0.296307034174820682626005918791634030640125274658203125;-0.04292926070828888274188983587009715847671031951904296875;-0.223206488706550632006297973930486477911472320556640625;-0.70255966668260316776439822206157259643077850341796875]
      mask Display: e = 0.06;c1 = [120 150 230]/255;c2 = ([120 150 230]+0)/383;c3 = ([120 150 230]+128)/383;patch([0 1 1 0],[0 0 1 1],c1);patch([0 1 1 1-e 1-e 0+e],[0 0 1 1-e 0+e 0+e],c2);patch([0 0 1 1-e 0+e 0+e],[0 1 1 1-e 1-e 0+e],c3);plot([0 1 1 0 0],[0 0 1 1 0]);disp('Weights');
  "IW{1,1}(9,:)'" : Constant  Value=[0.71564094376930054153262972249649465084075927734375;-0.66643746606927523057350981616764329373836517333984375;-1.1876237171727679342581041055382229387760162353515625;-1.1382882243704444125143027122248895466327667236328125;-0.0809094560829008713209731240567634813487529754638671875;-0.840593225903782492736127096577547490596771240234375;0.5717505543374763465891419400577433407306671142578125;-0.1284667707018977977906359910775790922343730926513671875;-0.09681800488201751375694215084877214394509792327880859375;-0.191492585246905544504869567390414886176586151123046875]
      mask Display: e = 0.06;c1 = [120 150 230]/255;c2 = ([120 150 230]+0)/383;c3 = ([120 150 230]+128)/383;patch([0 1 1 0],[0 0 1 1],c1);patch([0 1 1 1-e 1-e 0+e],[0 0 1 1-e 0+e 0+e],c2);patch([0 0 1 1-e 0+e 0+e],[0 1 1 1-e 1-e 0+e],c3);plot([0 1 1 0 0],[0 0 1 1 0]);disp('Weights');
  Mux : Mux  Inputs=40
      mask Display: e = 0.06;c1 = [120 150 230]/255;c2 = ([120 150 230]+0)/383;c3 = ([120 150 230]+128)/383;patch([0 1 1 0],[0 0 1 1],c1);patch([0 1 1 1-e 1-e 0+e],[0 0 1 1-e 0+e 0+e],c2);patch([0 0 1 1-e 0+e 0+e],[0 1 1 1-e 1-e 0+e],c3);plot([0 1 1 0 0],[0 0 1 1 0]);disp('Mux');
  dotprod{1..40} (40 alike) : neural/Weight Functions/dotprod
  "iz{1,1}" : Outport
      mask Display: e = 0.06;c1 = [120 230 180]/255;c2 = ([120 230 180]+0)/(256+128);c3 = ([120 230 180]+128)/(256+128);patch([0 1 1 0],[0 0 1 1],c1);patch([0 1 1 1-e 1-e 0+e],[0 0 1 1-e 0+e 0+e],c2);patch([0 0 1 1-e 0+e 0+e],[0 1 1 1-e 1-e 0+e],c3);plot([0 1 1 0 0],[0 0 1 1 0]);
  wires:
  "IW{1,1}(1,:)'"/1 -> dotprod1/1
  "pd{1,1}"/1 -> dotprod1/2, dotprod2/2, dotprod3/2, dotprod4/2, dotprod5/2, dotprod6/2, dotprod7/2, dotprod8/2, dotprod9/2, dotprod10/2, dotprod11/2, dotprod12/2, dotprod13/2, dotprod14/2, dotprod15/2, dotprod16/2, dotprod17/2, dotprod18/2, dotprod19/2, dotprod20/2, dotprod21/2, dotprod22/2, dotprod23/2, dotprod24/2, dotprod25/2, dotprod26/2, dotprod27/2, dotprod28/2, dotprod29/2, dotprod30/2, dotprod31/2, dotprod32/2, dotprod33/2, dotprod34/2, dotprod35/2, dotprod36/2, dotprod37/2, dotprod38/2, dotprod39/2, dotprod40/2
  dotprod1/1 -> Mux/1
  "IW{1,1}(2,:)'"/1 -> dotprod2/1
  dotprod2/1 -> Mux/2
  "IW{1,1}(3,:)'"/1 -> dotprod3/1
  dotprod3/1 -> Mux/3
  "IW{1,1}(4,:)'"/1 -> dotprod4/1
  dotprod4/1 -> Mux/4
  "IW{1,1}(5,:)'"/1 -> dotprod5/1
  dotprod5/1 -> Mux/5
  "IW{1,1}(6,:)'"/1 -> dotprod6/1
  dotprod6/1 -> Mux/6
  "IW{1,1}(7,:)'"/1 -> dotprod7/1
  dotprod7/1 -> Mux/7
  "IW{1,1}(8,:)'"/1 -> dotprod8/1
  dotprod8/1 -> Mux/8
  "IW{1,1}(9,:)'"/1 -> dotprod9/1
  dotprod9/1 -> Mux/9
  "IW{1,1}(10,:)'"/1 -> dotprod10/1
  dotprod10/1 -> Mux/10
  "IW{1,1}(11,:)'"/1 -> dotprod11/1
  dotprod11/1 -> Mux/11
  "IW{1,1}(12,:)'"/1 -> dotprod12/1
  dotprod12/1 -> Mux/12
  "IW{1,1}(13,:)'"/1 -> dotprod13/1
  dotprod13/1 -> Mux/13
  "IW{1,1}(14,:)'"/1 -> dotprod14/1
  dotprod14/1 -> Mux/14
  "IW{1,1}(15,:)'"/1 -> dotprod15/1
  dotprod15/1 -> Mux/15
  "IW{1,1}(16,:)'"/1 -> dotprod16/1
  dotprod16/1 -> Mux/16
  "IW{1,1}(17,:)'"/1 -> dotprod17/1
  dotprod17/1 -> Mux/17
  "IW{1,1}(18,:)'"/1 -> dotprod18/1
  dotprod18/1 -> Mux/18
  "IW{1,1}(19,:)'"/1 -> dotprod19/1
  dotprod19/1 -> Mux/19
  "IW{1,1}(20,:)'"/1 -> dotprod20/1
  dotprod20/1 -> Mux/20
  "IW{1,1}(21,:)'"/1 -> dotprod21/1
  dotprod21/1 -> Mux/21
  "IW{1,1}(22,:)'"/1 -> dotprod22/1
  dotprod22/1 -> Mux/22
  "IW{1,1}(23,:)'"/1 -> dotprod23/1
  dotprod23/1 -> Mux/23
  "IW{1,1}(24,:)'"/1 -> dotprod24/1
  dotprod24/1 -> Mux/24
  "IW{1,1}(25,:)'"/1 -> dotprod25/1
  dotprod25/1 -> Mux/25
  "IW{1,1}(26,:)'"/1 -> dotprod26/1
  dotprod26/1 -> Mux/26
  "IW{1,1}(27,:)'"/1 -> dotprod27/1
  dotprod27/1 -> Mux/27
  "IW{1,1}(28,:)'"/1 -> dotprod28/1
  dotprod28/1 -> Mux/28
  "IW{1,1}(29,:)'"/1 -> dotprod29/1
  dotprod29/1 -> Mux/29
  "IW{1,1}(30,:)'"/1 -> dotprod30/1
  dotprod30/1 -> Mux/30
  "IW{1,1}(31,:)'"/1 -> dotprod31/1
  dotprod31/1 -> Mux/31
  "IW{1,1}(32,:)'"/1 -> dotprod32/1
  dotprod32/1 -> Mux/32
  "IW{1,1}(33,:)'"/1 -> dotprod33/1
  dotprod33/1 -> Mux/33
  "IW{1,1}(34,:)'"/1 -> dotprod34/1
  dotprod34/1 -> Mux/34
  "IW{1,1}(35,:)'"/1 -> dotprod35/1
  dotprod35/1 -> Mux/35
  "IW{1,1}(36,:)'"/1 -> dotprod36/1
  dotprod36/1 -> Mux/36
  "IW{1,1}(37,:)'"/1 -> dotprod37/1
  dotprod37/1 -> Mux/37
  "IW{1,1}(38,:)'"/1 -> dotprod38/1
  dotprod38/1 -> Mux/38
  "IW{1,1}(39,:)'"/1 -> dotprod39/1
  dotprod39/1 -> Mux/39
  "IW{1,1}(40,:)'"/1 -> dotprod40/1
  dotprod40/1 -> Mux/40
  Mux/1 -> "iz{1,1}"/1

== system mrefrobotarm_modified_previous_y_previous_u_previous_ref_Thao/trimmed_cex_2/Layer 2/Delays 1 ==
  "p{2}" : Inport  PortDimensions=40
      mask Display: e = 0.06;c1 = [120 230 180]/255;c2 = ([120 230 180]+0)/(256+128);c3 = ([120 230 180]+128)/(256+128);patch([0 1 1 0],[0 0 1 1],c1);patch([0 1 1 1-e 1-e 0+e],[0 0 1 1-e 0+e 0+e],c2);patch([0 0 1 1-e 0+e 0+e],[0 1 1 1-e 1-e 0+e],c3);plot([0 1 1 0 0],[0 0 1 1 0]);
  mux : Mux  Inputs=1
      mask Display: e = 0.06;c1 = [120 150 230]/255;c2 = ([120 150 230]+0)/383;c3 = ([120 150 230]+128)/383;patch([0 1 1 0],[0 0 1 1],c1);patch([0 1 1 1-e 1-e 0+e],[0 0 1 1-e 0+e 0+e],c2);patch([0 0 1 1-e 0+e 0+e],[0 1 1 1-e 1-e 0+e],c3);plot([0 1 1 0 0],[0 0 1 1 0]);disp('Mux')
  "pd{2,1}" : Outport
      mask Display: e = 0.06;c1 = [120 230 180]/255;c2 = ([120 230 180]+0)/(256+128);c3 = ([120 230 180]+128)/(256+128);patch([0 1 1 0],[0 0 1 1],c1);patch([0 1 1 1-e 1-e 0+e],[0 0 1 1-e 0+e 0+e],c2);patch([0 0 1 1-e 0+e 0+e],[0 1 1 1-e 1-e 0+e],c3);plot([0 1 1 0 0],[0 0 1 1 0]);
  wires:
  "p{2}"/1 -> mux/1
  mux/1 -> "pd{2,1}"/1

== system mrefrobotarm_modified_previous_y_previous_u_previous_ref_Thao/trimmed_cex_2/Layer 2/LW{2,1} ==
  "ad{2,1}" : Inport  PortDimensions=40
      mask Display: e = 0.06;c1 = [120 230 180]/255;c2 = ([120 230 180]+0)/(256+128);c3 = ([120 230 180]+128)/(256+128);patch([0 1 1 0],[0 0 1 1],c1);patch([0 1 1 1-e 1-e 0+e],[0 0 1 1-e 0+e 0+e],c2);patch([0 0 1 1-e 0+e 0+e],[0 1 1 1-e 1-e 0+e],c3);plot([0 1 1 0 0],[0 0 1 1 0]);
  "IW{2,1}(1,:)'" : Constant  Value=[-0.2426809349482803579434175844653509557247161865234375;0.025038231950387547508629637604826712049543857574462890625;0.25301140507332642304305636571370996534824371337890625;-0.4504173254410233084854553453624248504638671875;-0.401301366195814523951668206791509874165058135986328125;0.0348180234027976875932353095777216367423534393310546875;-0.001871225764898266051561304124106754898093640804290771484375;0.5711631527413256748104686266742646694183349609375;0.06425088469726909778945156404006411321461200714111328125;0.38316268485787841058254343806765973567962646484375;0.41275086635921554023553881052066572010517120361328125;0.977046744129719701987824009847827255725860595703125;0.9131281314410035765405382335302419960498809814453125;-0.6489750971821333092037775713833980262279510498046875;-0.259336078442426842816104226585594005882740020751953125;0.265880648935690022671707311019417829811573028564453125;-0.36654898555592152487037083119503222405910491943359375;0.6902052769126687525869101591524668037891387939453125;0.33529358244700901980905882737715728580951690673828125;0.94711860650246071369195988154388032853603363037109375;-0.01056123791864854548350205476481278310529887676239013671875;0.3021276209072587537463050466612912714481353759765625;0.53430243973286895009522368127363733947277069091796875;-0.42243982779031219454424217474297620356082916259765625;-0.52532342973253431939184565635514445602893829345703125;-0.30854396824034335811148821449023671448230743408203125;-0.453934565234010267698039342576521448791027069091796875;-0.25454361643597012143658275817870162427425384521484375;0.061081850565629279559143327560377656482160091400146484375;0.86727996913510019272308682047878392040729522705078125;0.402161305557995729653697480898699723184108734130859375;0.19338772904372536487471734290011227130889892578125;0.35543765632189394665374493342824280261993408203125;-0.269008219385541369472747419422375969588756561279296875;0.38289705465027046304982150104478932917118072509765625;-1.104964362040833147915463996469043195247650146484375;0.0350104850231500452917288157550501637160778045654296875;-0.426520517320195191590670447112643159925937652587890625;-0.11378943795528673188499624302494339644908905029296875;-0.05186535903445625705909804992188583128154277801513671875]
      mask Display: e = 0.06;c1 = [120 150 230]/255;c2 = ([120 150 230]+0)/383;c3 = ([120 150 230]+128)/383;patch([0 1 1 0],[0 0 1 1],c1);patch([0 1 1 1-e 1-e 0+e],[0 0 1 1-e 0+e 0+e],c2);patch([0 0 1 1-e 0+e 0+e],[0 1 1 1-e 1-e 0+e],c3);plot([0 1 1 0 0],[0 0 1 1 0]);disp('weights');
  Mux : Mux  Inputs=1
      mask Display: e = 0.06;c1 = [120 150 230]/255;c2 = ([120 150 230]+0)/383;c3 = ([120 150 230]+128)/383;patch([0 1 1 0],[0 0 1 1],c1);patch([0 1 1 1-e 1-e 0+e],[0 0 1 1-e 0+e 0+e],c2);patch([0 0 1 1-e 0+e 0+e],[0 1 1 1-e 1-e 0+e],c3);plot([0 1 1 0 0],[0 0 1 1 0]);disp('Mux');
  dotprod1 : neural/Weight Functions/dotprod
  "lz{2,1}" : Outport
      mask Display: e = 0.06;c1 = [120 230 180]/255;c2 = ([120 230 180]+0)/(256+128);c3 = ([120 230 180]+128)/(256+128);patch([0 1 1 0],[0 0 1 1],c1);patch([0 1 1 1-e 1-e 0+e],[0 0 1 1-e 0+e 0+e],c2);patch([0 0 1 1-e 0+e 0+e],[0 1 1 1-e 1-e 0+e],c3);plot([0 1 1 0 0],[0 0 1 1 0]);
  wires:
  "IW{2,1}(1,:)'"/1 -> dotprod1/1
  "ad{2,1}"/1 -> dotprod1/2
  dotprod1/1 -> Mux/1
  Mux/1 -> "lz{2,1}"/1
